simulink model "Model_3_equalLoadSharing_pic"  (R2024a)
settings: Solver=VariableStepAuto  StartTime=0.0  StopTime=10.0  RelTol=1e-3
libraries: spsSeriesRLCBranchLib x5, spsMosfetLib x4, spsDiodeLib x2, spsIGBTDiodeLib x2, slpidlib x2, spsPWMGeneratorDCDCLib x2, spsVoltageMeasurementLib x2, spsCurrentMeasurementLib x1, spsFuelCellStackLib x1, spsDCVoltageSourceLib x1, spsSinglePhaseAsynchronousMachineLib x1
settings Model: Creator=yashu  LastModifiedBy=yashu

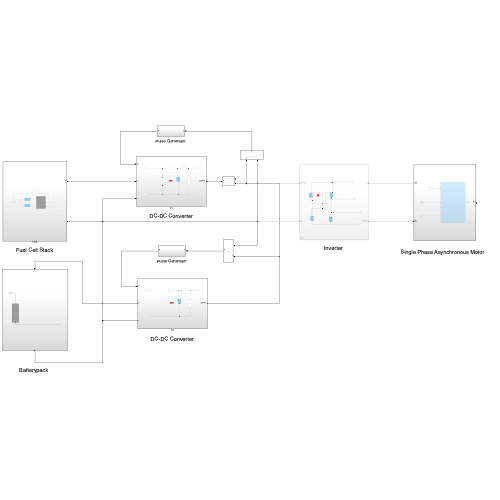
[thumbnail: Simulink's stored preview of the top-level diagram]
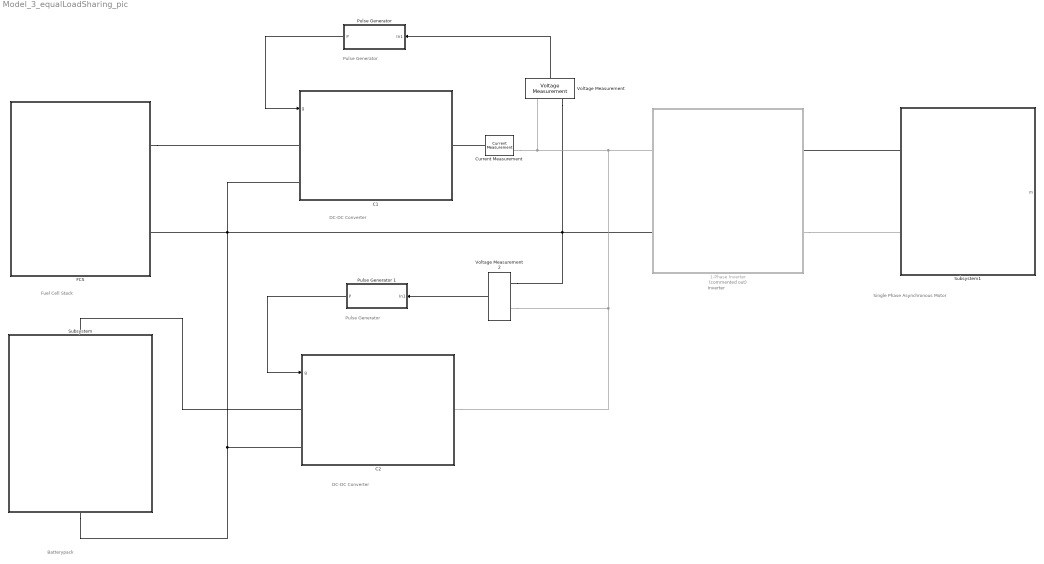
== system Model_3_equalLoadSharing_pic ==
  note: Fuel Cell Stack
  note: DC-DC Converter
  note: Inverter
  note: Pulse Generator
  note: Batterypack
  note: Single Phase Asynchronous Motor
  note: DC-DC Converter
  note: Pulse Generator
  1-Phase Inverter : Subsystem  Commented=on
  C1 : Subsystem
  C2 : Subsystem
  Current Measurement : spsCurrentMeasurementLib/Current Measurement  PhasorSimulation=off  OutputType=Complex  PSBequivalent=0
  FCS : Subsystem
  "Pulse Generator " : Subsystem
  Pulse Generator 1 : Subsystem
  Subsystem : Subsystem
  Subsystem1 : Subsystem
  Voltage Measurement : spsVoltageMeasurementLib/Voltage Measurement  PhasorSimulation=off  OutputType=Complex  PSBequivalent=0
  Voltage Measurement2 : spsVoltageMeasurementLib/Voltage Measurement  PhasorSimulation=off  OutputType=Complex  PSBequivalent=0
  wires:
  "Pulse Generator "/1(P) -> C1/1(g)
  Voltage Measurement/1 -> "Pulse Generator "/1(In1)
  Voltage Measurement2/1 -> Pulse Generator 1/1(In1)
  Pulse Generator 1/1(P) -> C2/1(g)
  connections:
  Subsystem/LConn1 -- C2/LConn2 -- 1-Phase Inverter/LConn2 -- Voltage Measurement2/LConn2 -- Voltage Measurement/LConn2 -- C1/LConn2 -- FCS/RConn2
  1-Phase Inverter/LConn1 -- Current Measurement/RConn1 -- Voltage Measurement/LConn1 -- C2/RConn1 -- Voltage Measurement2/LConn1
  1-Phase Inverter/RConn2 -- Subsystem1/LConn2
  FCS/RConn1 -- C1/LConn1
  Subsystem/RConn1 -- C2/LConn1
  Current Measurement/LConn1 -- C1/RConn1
  Subsystem1/LConn1 -- 1-Phase Inverter/RConn1

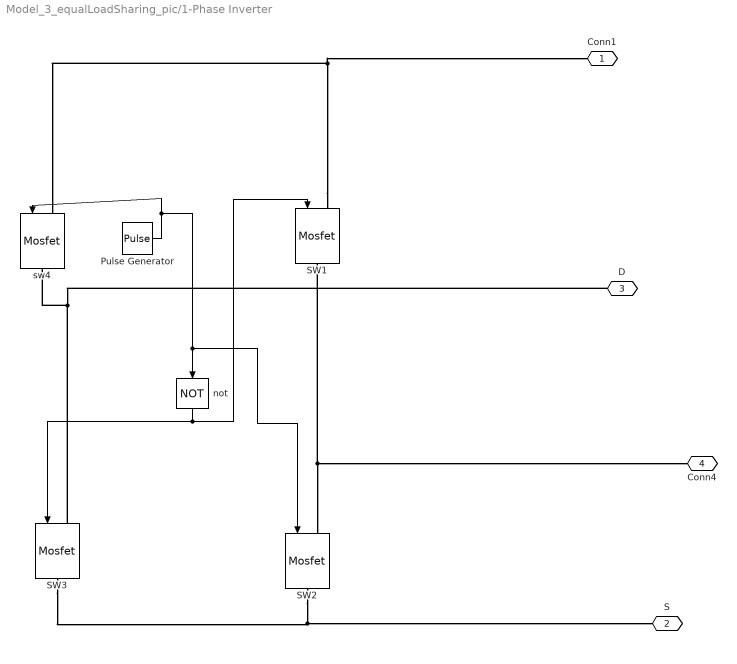
== system Model_3_equalLoadSharing_pic/1-Phase Inverter ==
  "  SW2   " : spsMosfetLib/Mosfet  Ron=0.1  Lon=0  Rd=0.01  Vfd=0  IC=0  Rs=1e5  Cs=inf  Measurements=off
  " SW3   " : spsMosfetLib/Mosfet  Ron=0.1  Lon=0  Rd=0.01  Vfd=0  IC=0  Rs=1e5  Cs=inf  Measurements=off
  " sw4   " : spsMosfetLib/Mosfet  Ron=0.1  Lon=0  Rd=0.01  Vfd=0  IC=0  Rs=1e5  Cs=inf  Measurements=off
  Pulse Generator : DiscretePulseGenerator  PulseType=Time based  Period=20e-3  PulseWidth=50
  "SW1    " : spsMosfetLib/Mosfet  Ron=0.1  Lon=0  Rd=0.01  Vfd=0  IC=0  Rs=1e5  Cs=inf  Measurements=off
  not : Logic  Operator=NOT  AllPortsSameDT=off  OutDataTypeStr=boolean
  Conn1 : PMIOPort  Side=Left
  S : PMIOPort  Port=2  Side=Left
  D : PMIOPort  Port=3  Side=Right
  Conn4 : PMIOPort  Port=4  Side=Right
  wires:
  not/1 -> " SW3   "/1, "SW1    "/1
  Pulse Generator/1 -> " sw4   "/1, "  SW2   "/1, not/1
  connections:
  " sw4   "/RConn1 -- D/RConn1 -- " SW3   "/LConn1
  " SW3   "/RConn1 -- "  SW2   "/RConn1 -- S/RConn1
  "SW1    "/RConn1 -- Conn4/RConn1 -- "  SW2   "/LConn1
  "SW1    "/LConn1 -- " sw4   "/LConn1 -- Conn1/RConn1

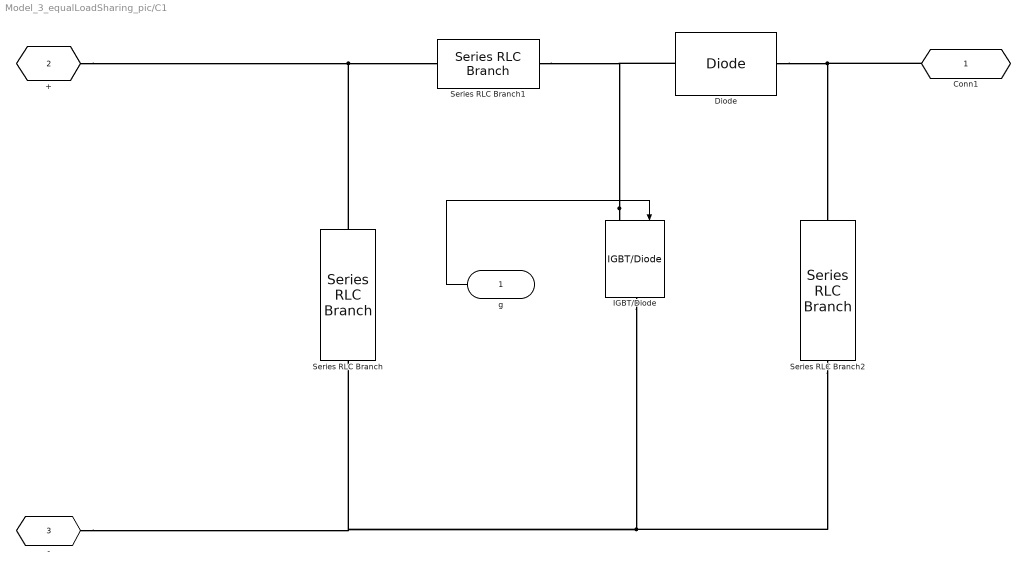
== system Model_3_equalLoadSharing_pic/C1 ==
  g : Inport
  Diode : spsDiodeLib/Diode  Ron=0.001  Lon=0  Vf=0.8  IC=0  UseSnubber=0  Rs=500  Cs=250e-9  Measurements=off
  IGBT/Diode : spsIGBTDiodeLib/IGBT//Diode  Ron=1e-3  Rs=1e5  Cs=inf  Measurements=off
  Series RLC Branch : spsSeriesRLCBranchLib/Series RLC Branch  LConnTagsString=__new0  RConnTagsString=__new0  BranchType=C  Resistance=1  Inductance=1e-3  SetiL0=off  InitialCurrent=0  Capacitance=0.00035  Setx0=off  InitialVoltage=0  Measurements=None
  Series RLC Branch1 : spsSeriesRLCBranchLib/Series RLC Branch  LConnTagsString=__new0  RConnTagsString=__new0  BranchType=L  Resistance=1  Inductance=0.0018  SetiL0=off  InitialCurrent=0  Capacitance=1e-6  Setx0=off  InitialVoltage=0  Measurements=None
  Series RLC Branch2 : spsSeriesRLCBranchLib/Series RLC Branch  LConnTagsString=__new0  RConnTagsString=__new0  BranchType=C  Resistance=1  Inductance=1e-3  SetiL0=off  InitialCurrent=0  Capacitance=0.00035  Setx0=off  InitialVoltage=0  Measurements=None
  Conn1 : PMIOPort  Side=Right
  + : PMIOPort  Port=2  Side=Left
  - : PMIOPort  Port=3  Side=Left
  wires:
  g/1 -> IGBT/Diode/1
  connections:
  IGBT/Diode/LConn1 -- Series RLC Branch1/RConn1 -- Diode/LConn1
  Diode/RConn1 -- Series RLC Branch2/LConn1 -- Conn1/RConn1
  Series RLC Branch2/RConn1 -- -/RConn1 -- Series RLC Branch/RConn1 -- IGBT/Diode/RConn1
  Series RLC Branch/LConn1 -- +/RConn1 -- Series RLC Branch1/LConn1

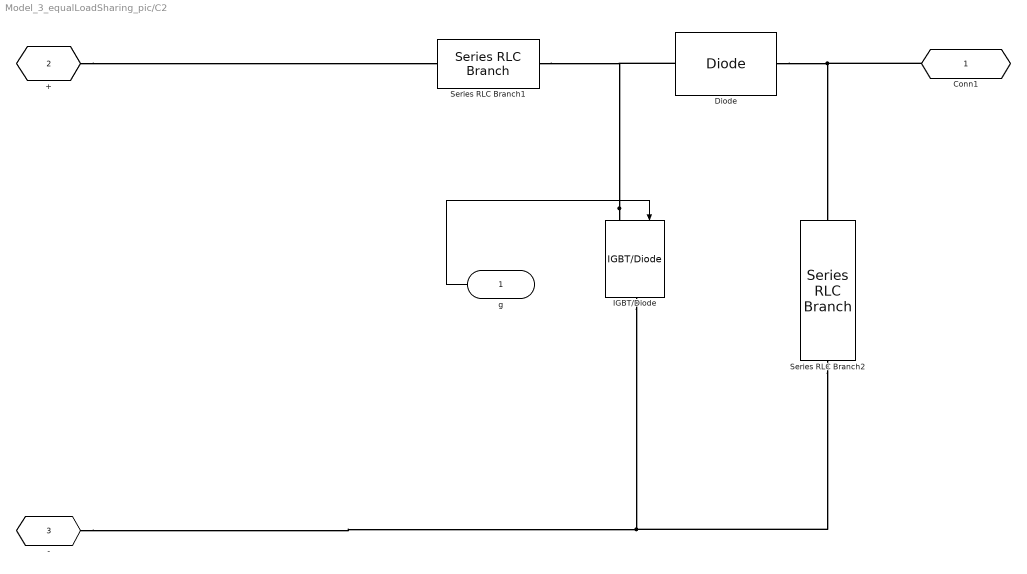
== system Model_3_equalLoadSharing_pic/C2 ==
  g : Inport
  Diode : spsDiodeLib/Diode  Ron=0.001  Lon=0  Vf=0.8  IC=0  UseSnubber=0  Rs=500  Cs=250e-9  Measurements=off
  IGBT/Diode : spsIGBTDiodeLib/IGBT//Diode  Ron=1e-3  Rs=1e5  Cs=inf  Measurements=off
  Series RLC Branch1 : spsSeriesRLCBranchLib/Series RLC Branch  LConnTagsString=__new0  RConnTagsString=__new0  BranchType=L  Resistance=1  Inductance=0.00114  SetiL0=off  InitialCurrent=0  Capacitance=1e-6  Setx0=off  InitialVoltage=0  Measurements=None
  Series RLC Branch2 : spsSeriesRLCBranchLib/Series RLC Branch  LConnTagsString=__new0  RConnTagsString=__new0  BranchType=C  Resistance=1  Inductance=1e-3  SetiL0=off  InitialCurrent=0  Capacitance=0.000215  Setx0=off  InitialVoltage=0  Measurements=None
  Conn1 : PMIOPort  Side=Right
  + : PMIOPort  Port=2  Side=Left
  - : PMIOPort  Port=3  Side=Left
  wires:
  g/1 -> IGBT/Diode/1
  connections:
  IGBT/Diode/LConn1 -- Series RLC Branch1/RConn1 -- Diode/LConn1
  Diode/RConn1 -- Series RLC Branch2/LConn1 -- Conn1/RConn1
  Series RLC Branch2/RConn1 -- -/RConn1 -- IGBT/Diode/RConn1
  +/RConn1 -- Series RLC Branch1/LConn1

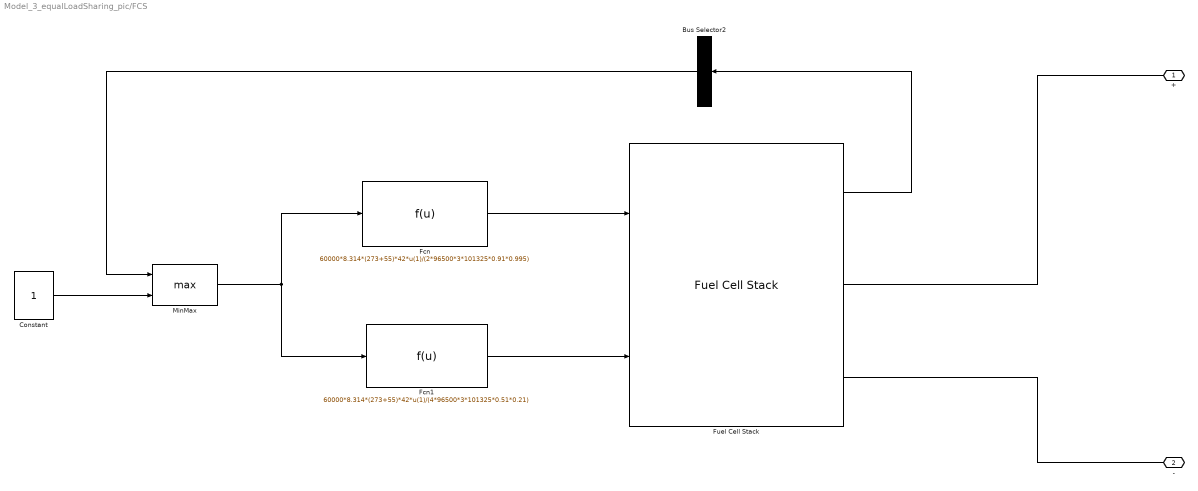
== system Model_3_equalLoadSharing_pic/FCS ==
  Bus Selector2 : BusSelector  OutputSignals=Current  OutputAsBus=on
  Constant : Constant
  Fcn : Fcn  Expr=60000*8.314*(273+55)*42*u(1)/(2*96500*3*101325*0.91*0.995)
  Fcn1 : Fcn  Expr=60000*8.314*(273+55)*42*u(1)/(4*96500*3*101325*0.51*0.21)
  Fuel Cell Stack : spsFuelCellStackLib/Fuel Cell Stack  PresetModel=PEMFC - 1.26 kW - 24 Vdc  FcType=0  Detailed=Detailed  Eoc=[42,35]  NomVI=[52,24.23]  EndVI=[100,20]  Nc=42  n=46  TOp=55  AirFr=2400  SuppPress=[1.5,1]  Comp=[99.95,21,1]  SignX=off  SignY=off  FlowRateH2=on  FlowRateAir=on  SystemTemp=off  SystemPH2=off  SystemPAir=off  FCDyn=off  FC_tau=1  Peak_O2=80  V_Under=10
      settings: LibrarySourceBlock=sps_lib/Sources/Fuel Cell Stack
  MinMax : MinMax  Function=max  Inputs=2
  + : PMIOPort  Side=Right
  - : PMIOPort  Port=2  Side=Right
  wires:
  Fuel Cell Stack/1 -> Bus Selector2/1
  Fcn1/1 -> Fuel Cell Stack/2
  MinMax/1 -> Fcn/1, Fcn1/1
  Constant/1 -> MinMax/2
  Fcn/1 -> Fuel Cell Stack/1
  Bus Selector2/1 -> MinMax/1
  connections:
  Fuel Cell Stack/RConn1 -- +/RConn1
  -/RConn1 -- Fuel Cell Stack/RConn2

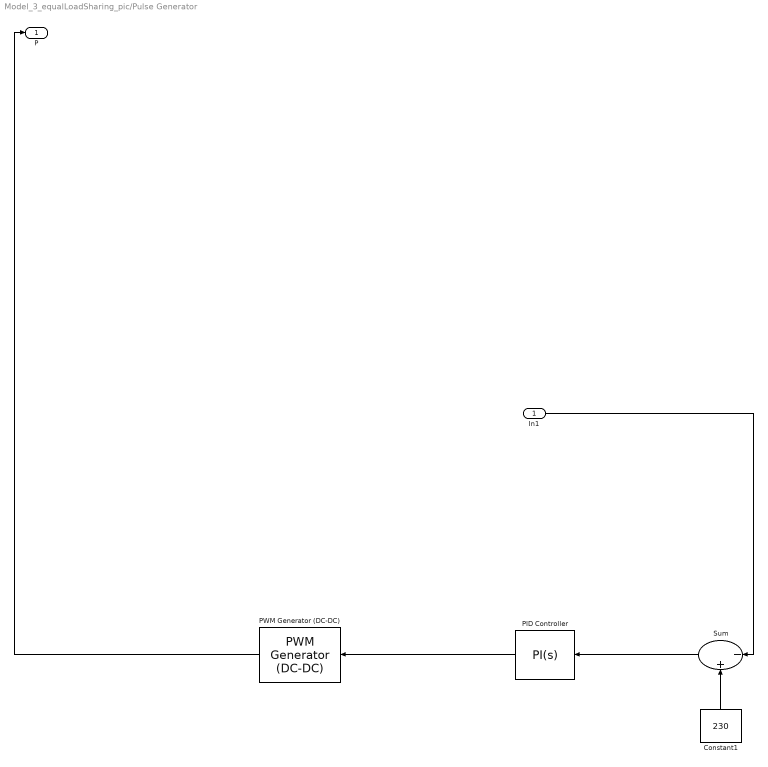
== system Model_3_equalLoadSharing_pic/Pulse Generator  ==
  In1 : Inport
  Constant1 : Constant  Value=230
  PID Controller : slpidlib/PID Controller  Controller=PI  Form=Parallel  TimeDomain=Continuous-time  UseExternalTs=off  SampleTime=-1  IntegratorMethod=Forward Euler  FilterMethod=Forward Euler  ControllerParametersSource=internal  P=0  I=0.02  UseKiTs=off  D=0  UseExternalDerivativeSource=off  N=100  UseFilter=on  TunerSelectOption=Transfer Function Based (PID Tuner App)  InitialConditionSource=internal  InitialConditionForIntegrator=0  InitialConditionForFilter=0  DifferentiatorICPrevScaledInput=0  ExternalReset=none  TrackingMode=off  Kt=1  LimitOutput=off  SatLimitsSource=internal  UpperSaturationLimit=inf  LowerSaturationLimit=-inf  LinearizeAsGain=on  AntiWindupMode=none  Kb=1  LimitIntegrator=off  UpperIntegratorSaturationLimit=inf  LowerIntegratorSaturationLimit=-inf  POutMin=[]  POutMax=[]  IOutMin=[]  IOutMax=[]  DOutMin=[]  DOutMax=[]  NOutMin=[]  NOutMax=[]  SumOutMin=[]  SumOutMax=[]  SaturationOutMin=[]  SaturationOutMax=[]  PParamMin=[]  PParamMax=[]  IParamMin=[]  IParamMax=[]  DParamMin=[]  DParamMax=[]  NParamMin=[]  NParamMax=[]  KbParamMin=[]  KbParamMax=[]  KtParamMin=[]  KtParamMax=[]  KbOutMin=[]  KbOutMax=[]  KtOutMin=[]  KtOutMax=[]  IntegratorOutMin=[]  IntegratorOutMax=[]  FilterOutMin=[]  FilterOutMax=[]  SumI1OutMin=[]  SumI1OutMax=[]  SumI2OutMin=[]  SumI2OutMax=[]  SumI3OutMin=[]  SumI3OutMax=[]  SumI4OutMin=[]  SumI4OutMax=[]  SumDOutMin=[]  SumDOutMax=[]  DifferentiatorOutMin=[]  DifferentiatorOutMax=[]  FilterDiffOutCoefMin=[]  FilterDiffOutCoefMax=[]  ReciprocalOutMin=[]  ReciprocalOutMax=[]  SumDenOutMin=[]  SumDenOutMax=[]  SumNumOutMin=[]  SumNumOutMax=[]  DivideOutMin=[]  DivideOutMax=[]  UdiffTsProdOutMin=[]  UdiffTsProdOutMax=[]  NTsProdOutMin=[]  NTsProdOutMax=[]  UintegralTsProdOutMin=[]  UintegralTsProdOutMax=[]  UngainTsProdOutMin=[]  UngainTsProdOutMax=[]  ClampingZeroOutDataTypeStr=Inherit: Inherit via back propagation  ClampingZeroOutMin=[]  ClampingZeroOutMax=[]  FilterDenConstantOutDataTypeStr=Inherit: Inherit via back propagation  FilterDenConstantOutMin=[]  FilterDenConstantOutMax=[]  PCopyOutDataTypeStr=Inherit: Inherit via back propagation  PCopyOutMin=[]  PCopyOutMax=[]  NCopyOutDataTypeStr=Inherit: Inherit via back propagation  NCopyOutMin=[]  NCopyOutMax=[]  IntegratorContinuousStateAttributes=''  IntegratorStateMustResolveToSignalObject=off  IntegratorRTWStateStorageClass=Auto  FilterContinuousStateAttributes=''  FilterStateMustResolveToSignalObject=off  FilterRTWStateStorageClass=Auto  ParallelPVariant=InternalParameters  IdealPVariant=Disabled  IVariant=InternalParameters  DVariant=Disabled  IntegratorVariant=Continuous  SatVariant=Disabled  AWVariant=Passthrough  PCopyVariant=Disabled  TRVariant=Disabled  FdbkBlocksVariant=Forward  IdealPFdbkVariant=Disabled  SatFdbkVariant=Disabled  DerivativeFilterVariant=Disabled  NVariant=Disabled  NCopyVariant=Disabled_SignalSpec  FilterICVariant=Disabled  IntegratorICVariant=InternalICs  ExternalResetVariant=Disabled  TRSumVariant=Passthrough  SumFdbkVariant=Disabled  SumVariant=Sum_PI  TsampFilterVariant=InternalTs  TsampNgainVariant=Passthrough  TsampIntegralVariant=Disabled_SignalSpec  ExternalSaturationOutDataTypeStr=Inherit: Same as second input  DerivativeSourceVariant=Disabled
  PWM Generator (DC-DC) : spsPWMGeneratorDCDCLib/PWM Generator (DC-DC)  Fsw=10000  Ts=0
  Sum : Sum  Inputs=|-+
  P : Outport
  wires:
  In1/1 -> Sum/1
  PWM Generator (DC-DC)/1 -> P/1
  PID Controller/1 -> PWM Generator (DC-DC)/1
  Sum/1 -> PID Controller/1
  Constant1/1 -> Sum/2

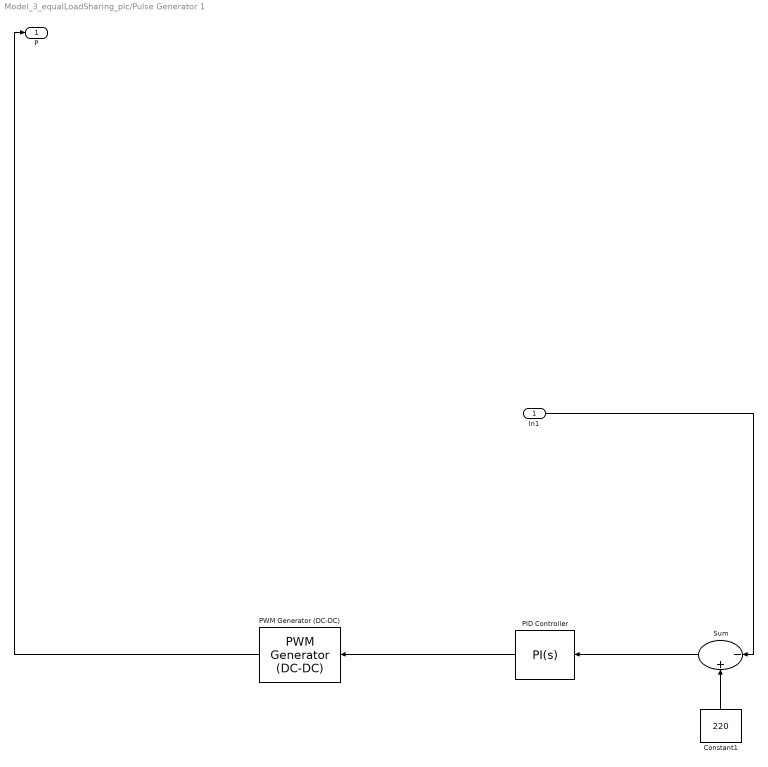
== system Model_3_equalLoadSharing_pic/Pulse Generator 1 ==
  In1 : Inport
  Constant1 : Constant  Value=220
  PID Controller : slpidlib/PID Controller  Controller=PI  Form=Parallel  TimeDomain=Continuous-time  UseExternalTs=off  SampleTime=-1  IntegratorMethod=Forward Euler  FilterMethod=Forward Euler  ControllerParametersSource=internal  P=0  I=0.02  UseKiTs=off  D=0  UseExternalDerivativeSource=off  N=100  UseFilter=on  TunerSelectOption=Transfer Function Based (PID Tuner App)  InitialConditionSource=internal  InitialConditionForIntegrator=0  InitialConditionForFilter=0  DifferentiatorICPrevScaledInput=0  ExternalReset=none  TrackingMode=off  Kt=1  LimitOutput=off  SatLimitsSource=internal  UpperSaturationLimit=inf  LowerSaturationLimit=-inf  LinearizeAsGain=on  AntiWindupMode=none  Kb=1  LimitIntegrator=off  UpperIntegratorSaturationLimit=inf  LowerIntegratorSaturationLimit=-inf  POutMin=[]  POutMax=[]  IOutMin=[]  IOutMax=[]  DOutMin=[]  DOutMax=[]  NOutMin=[]  NOutMax=[]  SumOutMin=[]  SumOutMax=[]  SaturationOutMin=[]  SaturationOutMax=[]  PParamMin=[]  PParamMax=[]  IParamMin=[]  IParamMax=[]  DParamMin=[]  DParamMax=[]  NParamMin=[]  NParamMax=[]  KbParamMin=[]  KbParamMax=[]  KtParamMin=[]  KtParamMax=[]  KbOutMin=[]  KbOutMax=[]  KtOutMin=[]  KtOutMax=[]  IntegratorOutMin=[]  IntegratorOutMax=[]  FilterOutMin=[]  FilterOutMax=[]  SumI1OutMin=[]  SumI1OutMax=[]  SumI2OutMin=[]  SumI2OutMax=[]  SumI3OutMin=[]  SumI3OutMax=[]  SumI4OutMin=[]  SumI4OutMax=[]  SumDOutMin=[]  SumDOutMax=[]  DifferentiatorOutMin=[]  DifferentiatorOutMax=[]  FilterDiffOutCoefMin=[]  FilterDiffOutCoefMax=[]  ReciprocalOutMin=[]  ReciprocalOutMax=[]  SumDenOutMin=[]  SumDenOutMax=[]  SumNumOutMin=[]  SumNumOutMax=[]  DivideOutMin=[]  DivideOutMax=[]  UdiffTsProdOutMin=[]  UdiffTsProdOutMax=[]  NTsProdOutMin=[]  NTsProdOutMax=[]  UintegralTsProdOutMin=[]  UintegralTsProdOutMax=[]  UngainTsProdOutMin=[]  UngainTsProdOutMax=[]  ClampingZeroOutDataTypeStr=Inherit: Inherit via back propagation  ClampingZeroOutMin=[]  ClampingZeroOutMax=[]  FilterDenConstantOutDataTypeStr=Inherit: Inherit via back propagation  FilterDenConstantOutMin=[]  FilterDenConstantOutMax=[]  PCopyOutDataTypeStr=Inherit: Inherit via back propagation  PCopyOutMin=[]  PCopyOutMax=[]  NCopyOutDataTypeStr=Inherit: Inherit via back propagation  NCopyOutMin=[]  NCopyOutMax=[]  IntegratorContinuousStateAttributes=''  IntegratorStateMustResolveToSignalObject=off  IntegratorRTWStateStorageClass=Auto  FilterContinuousStateAttributes=''  FilterStateMustResolveToSignalObject=off  FilterRTWStateStorageClass=Auto  ParallelPVariant=InternalParameters  IdealPVariant=Disabled  IVariant=InternalParameters  DVariant=Disabled  IntegratorVariant=Continuous  SatVariant=Disabled  AWVariant=Passthrough  PCopyVariant=Disabled  TRVariant=Disabled  FdbkBlocksVariant=Forward  IdealPFdbkVariant=Disabled  SatFdbkVariant=Disabled  DerivativeFilterVariant=Disabled  NVariant=Disabled  NCopyVariant=Disabled_SignalSpec  FilterICVariant=Disabled  IntegratorICVariant=InternalICs  ExternalResetVariant=Disabled  TRSumVariant=Passthrough  SumFdbkVariant=Disabled  SumVariant=Sum_PI  TsampFilterVariant=InternalTs  TsampNgainVariant=Passthrough  TsampIntegralVariant=Disabled_SignalSpec  ExternalSaturationOutDataTypeStr=Inherit: Same as second input  DerivativeSourceVariant=Disabled
  PWM Generator (DC-DC) : spsPWMGeneratorDCDCLib/PWM Generator (DC-DC)  Fsw=10000  Ts=0
  Sum : Sum  Inputs=|-+
  P : Outport
  wires:
  In1/1 -> Sum/1
  PWM Generator (DC-DC)/1 -> P/1
  PID Controller/1 -> PWM Generator (DC-DC)/1
  Sum/1 -> PID Controller/1
  Constant1/1 -> Sum/2

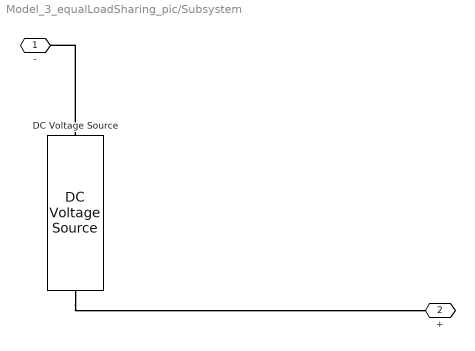
== system Model_3_equalLoadSharing_pic/Subsystem ==
  DC Voltage Source : spsDCVoltageSourceLib/DC Voltage Source  Amplitude=12  Measurements=None
  - : PMIOPort  Side=Left
  + : PMIOPort  Port=2  Side=Right
  connections:
  DC Voltage Source/LConn1 -- -/RConn1
  DC Voltage Source/RConn1 -- +/RConn1

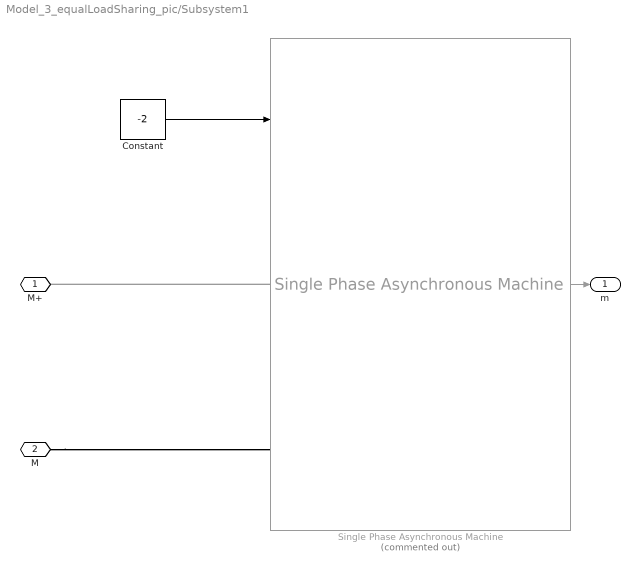
== system Model_3_equalLoadSharing_pic/Subsystem1 ==
  Constant : Constant  Value=-2
  Single Phase Asynchronous Machine : spsSinglePhaseAsynchronousMachineLib/Single Phase Asynchronous Machine  Commented=on  MechanicalLoad=Torque Tm  UNITS=SI  MachineType=Split Phase  MeasurementBus=off  NominalParameters="[ 1100 230  50]"  MainWindingStator=[2.02 0.0074]  MainWindingRotor=[4.12 0.0056001]  MutualInductance=0.17719  AuxiliaryWinding=[7.14 0.0085001]  Mechanical=[0.0146 0 2 1.18]  CapacitorStart=[2 0.0002547]  CapacitorRun=[18 2.11e-05]  DisconnectionSpeed=75  InitialSpeed=0  DataType=SI  TsPowergui=0  TsBlock=-1
      settings: LibrarySourceBlock=|
      | sps_lib/Electrical Machines/Single Phase
      | Asynchronous Machine
  M+ : PMIOPort  Side=Left
  M : PMIOPort  Port=2  Side=Left
  m : Outport
  wires:
  Single Phase Asynchronous Machine/1 -> m/1
  Constant/1 -> Single Phase Asynchronous Machine/1
  connections:
  M/RConn1 -- Single Phase Asynchronous Machine/LConn2
  Single Phase Asynchronous Machine/LConn1 -- M+/RConn1
